simulink model "sim_BTMS"  (R2022b)
settings: Solver=FixedStepAuto  StartTime=0.0  StopTime=SimPara.t_sim  FixedStep=0.001  RelTol=1e-3
values from neighbouring files (symbols this model uses):
  BatPara = get_BatPara(BatPara, config_battery)    [sim_BTMS_interface.m]
  p = epe_mod(jj).p    [main_sim_BTMS_1_system_setup.m]
  SysPara = rmfield(SysPara, {'p','s'})    [main_sim_BTMS_1_system_setup.m]
undefined symbols (not defined in the file or in its folder): A, BTMSConfig, i, LSAPara, SimPara, x2_cal, x3_cal, x_cal
libraries: simulink x14, dspstat3 x7, dspindex x1
(part 3 of 4)

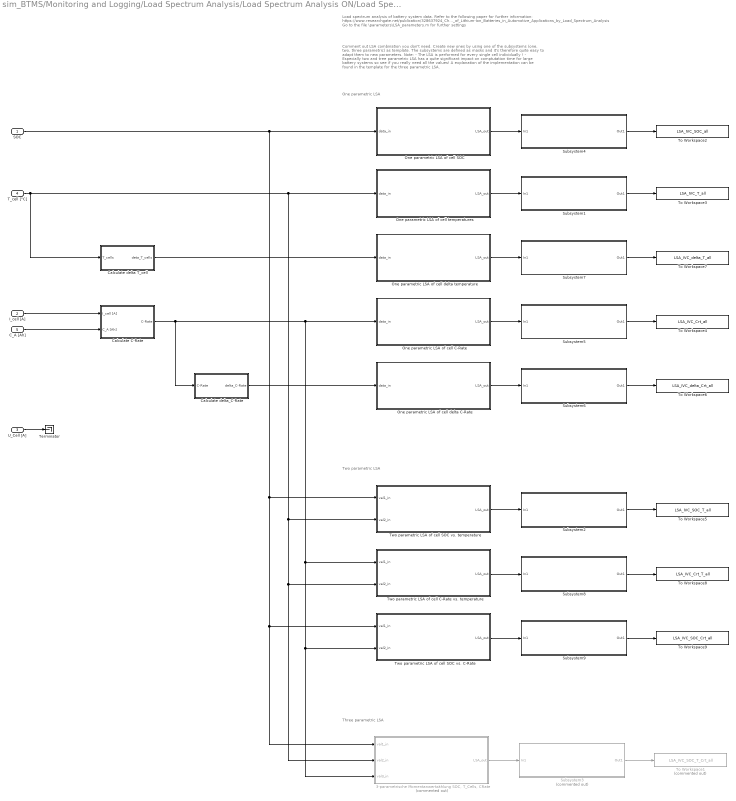
== system sim_BTMS/Monitoring and Logging/Load Spectrum Analysis/Load Spectrum Analysis ON/Load Spectrum Analysis ON ==
  note: Comment out LSA combination you don't need. Create new ones by using one of the subsystems (one, two, three parametric) as template. The subsystems are defined as masks
      | and it's therefore quite easy to adapt them to new parameters.
      |
      | Note:
      | - The LSA is performed for every single cell individually !
      | - Especially two and tree parametric LSA has a quite significant impact on comptutation time for large battery systems so see if you really need all the values!
      |
      | A explanation of the implementation can be found in the template for the three parametric LSA.
  note: Three parametric LSA
  note: Two parametric LSA
  note: One parametric LSA
  note: Load spectrum analysis of battery system data. Refer to the following paper for further information:
      | https://www.researchgate.net/publication/328637924_Characterization_and_Concept_Validation_of_Lithium-Ion_Batteries_in_Automotive_Applications_by_Load_Spectrum_Analysis
      |
      | Go to the file \parameters\LSA_parameters.m for further settings
  SOC : Inport
  I_cell [A] : Inport  Port=2
  U_Cell [A] : Inport  Port=3
  T_cell [°C] : Inport  Port=4
  C_A [Ah] : Inport  Port=5
  "3-parametrische Momentanwertzählung SOC, T_Cells, CRate" : Subsystem  Commented=on  mask{bins_borders_1=LSAPara.bins_borders_SOC, bins_mean_1=LSAPara.bins_mean_SOC, bins_borders_2=LSAPara.bins_borders_T, bins_mean_2=LSAPara.bins_mean_T, bins_borders_3=LSAPara.bins_borders_Crt, bins_mean_3=LSAPara.bins_mean_Crt}
      mask prompts: bins_borders_1 "Provide 'bins_borders'"; bins_mean_1 "Provide 'bins_mean'"; bins_borders_2 "Provide 'bins_borders'"; bins_mean_2 "Provide 'bins_mean'"; bins_borders_3 "Provide 'bins_borders'"; bins_mean_3 "Provide 'bins_mean'"
      mask DialogControl DescTextVar Prompt: Subsystem for three-parametric instantaneous value counting. Change the parameters below to select other system variables. Refer to parameters\LSA_parameters.m for further options.
      mask DialogControl Control2 Prompt: Copy&Paste this subsystem and double click to edit the variable assignments to monitor further variables.
      mask DialogControl Control3 Prompt: First system variable ('val 1')
      mask DialogControl Control4 Prompt: First system variable ('val 2')
      mask DialogControl Control5 Prompt: First system variable ('val 3')
      mask Display:
      | fprintf('Three parametric\ninstantaneous value\ncounting')
      | port_label('output', 1, 'load spectrum')
      | port_label('input', 1, 'timeseries val 1')
      | port_label('input', 2, 'timeseries val 2')
      | port_label('input', 3, 'timeseries val 3')
  Calculate C-Rate : Subsystem
  Calculate delta T_cell : Subsystem
  Calculate delta_C-Rate : Subsystem
  One parametric LSA of cell C-Rate : Subsystem  mask{bins_borders=LSAPara.bins_borders_Crt, bins_mean=LSAPara.bins_mean_Crt}
      mask prompts: bins_borders "Provide 'bins_borders'"; bins_mean "Provide 'bins_mean'"
      mask DialogControl DescTextVar Prompt: Subsystem for one-parametric instantaneous value counting. Change the parameters below to select other system variables. Refer to parameters\LSA_parameters.m for further options.
      mask DialogControl Control2 Prompt: Copy&Paste this subsystem and double click to edit the variable assignments to monitor further variables.
      mask Display:
      | fprintf('One parametric\ninstantaneous value\ncounting')
      | port_label('output', 1, 'load spectrum')
      | port_label('input', 1, 'timeseries')
  One parametric LSA of cell SOC : Subsystem  mask{bins_borders=LSAPara.bins_borders_SOC, bins_mean=LSAPara.bins_mean_SOC}
      mask prompts: bins_borders "Provide 'bins_borders'"; bins_mean "Provide 'bins_mean'"
      mask DialogControl DescTextVar Prompt: Subsystem for one-parametric instantaneous value counting. Change the parameters below to select other system variables. Refer to parameters\LSA_parameters.m for further options.
      mask DialogControl Control2 Prompt: Copy&Paste this subsystem and double click to edit the variable assignments to monitor further variables.
      mask Display:
      | fprintf('One parametric\ninstantaneous value\ncounting')
      | port_label('output', 1, 'load spectrum')
      | port_label('input', 1, 'timeseries')
  One parametric LSA of cell delta C-Rate : Subsystem  mask{bins_borders=LSAPara.bins_borders_delta_Crt, bins_mean=LSAPara.bins_mean_delta_Crt}
      mask prompts: bins_borders "Provide 'bins_borders'"; bins_mean "Provide 'bins_mean'"
      mask DialogControl DescTextVar Prompt: Subsystem for one-parametric instantaneous value counting. Change the parameters below to select other system variables. Refer to parameters\LSA_parameters.m for further options.
      mask DialogControl Control2 Prompt: Copy&Paste this subsystem and double click to edit the variable assignments to monitor further variables.
      mask Display:
      | fprintf('One parametric\ninstantaneous value\ncounting')
      | port_label('output', 1, 'load spectrum')
      | port_label('input', 1, 'timeseries')
  One parametric LSA of cell delta temperature : Subsystem  mask{bins_borders=LSAPara.bins_borders_delta_T, bins_mean=LSAPara.bins_mean_delta_T}
      mask prompts: bins_borders "Provide 'bins_borders'"; bins_mean "Provide 'bins_mean'"
      mask DialogControl DescTextVar Prompt: Subsystem for one-parametric instantaneous value counting. Change the parameters below to select other system variables. Refer to parameters\LSA_parameters.m for further options.
      mask DialogControl Control2 Prompt: Copy&Paste this subsystem and double click to edit the variable assignments to monitor further variables.
      mask Display:
      | fprintf('One parametric\ninstantaneous value\ncounting')
      | port_label('output', 1, 'load spectrum')
      | port_label('input', 1, 'timeseries')
  One parametric LSA of cell temperatures : Subsystem  mask{bins_borders=LSAPara.bins_borders_T, bins_mean=LSAPara.bins_mean_T}
      mask prompts: bins_borders "Provide 'bins_borders'"; bins_mean "Provide 'bins_mean'"
      mask DialogControl DescTextVar Prompt: Subsystem for one-parametric instantaneous value counting. Change the parameters below to select other system variables. Refer to parameters\LSA_parameters.m for further options.
      mask DialogControl Control2 Prompt: Copy&Paste this subsystem and double click to edit the variable assignments to monitor further variables.
      mask Display:
      | fprintf('One parametric\ninstantaneous value\ncounting')
      | port_label('output', 1, 'load spectrum')
      | port_label('input', 1, 'timeseries')
  Subsystem1 : Subsystem  mask{dim=2, start=99}
      mask prompts: dim "Select dimension"; start "Start concatenation after x%"
      mask DialogControl DescTextVar Prompt: Create one load spectrum from all individual cells. By default the LSA blocks create one load spectrum for every individual cell. This block creates one load-spectrum for all cells.
      mask DialogControl Control2 Prompt: Select the dimension of the load spectum in the parameter below. This uses the following logic:
      mask DialogControl Control3 Prompt: One parametric LS: Select "2"
      mask DialogControl Control4 Prompt: Two parametric LS: Select "3"
      mask DialogControl Control5 Prompt: Three parametric LS: Select "4"
      mask DialogControl Control6 Prompt: Only the last value of the load spectrum matrix is relevant, so we don't want to make the concatenation every simulation step. Therefore the system is set to only start with the calculation after 99% of the simulation is finished. If you need another value edit ist below.
      mask Display:
      | fprintf('Summed LSA\nfrom all cells')
      | port_label('input', 1, 'cell-individual LSA')
      | port_label('output', 1, 'summed LSA')
  Subsystem2 : Subsystem  mask{dim=3, start=99}
      mask prompts: dim "Select dimension"; start "Start concatenation after x%"
      mask DialogControl DescTextVar Prompt: Create one load spectrum from all individual cells. By default the LSA blocks create one load spectrum for every individual cell. This block creates one load-spectrum for all cells.
      mask DialogControl Control2 Prompt: Select the dimension of the load spectum in the parameter below. This uses the following logic:
      mask DialogControl Control3 Prompt: One parametric LS: Select "2"
      mask DialogControl Control4 Prompt: Two parametric LS: Select "3"
      mask DialogControl Control5 Prompt: Three parametric LS: Select "4"
      mask DialogControl Control6 Prompt: Only the last value of the load spectrum matrix is relevant, so we don't want to make the concatenation every simulation step. Therefore the system is set to only start with the calculation after 99% of the simulation is finished. If you need another value edit ist below.
      mask Display:
      | fprintf('Summed LSA\nfrom all cells')
      | port_label('input', 1, 'cell-individual LSA')
      | port_label('output', 1, 'summed LSA')
  Subsystem3 : Subsystem  Commented=on  mask{dim=4, start=99}
      mask prompts: dim "Select dimension"; start "Start concatenation after x%"
      mask DialogControl DescTextVar Prompt: Create one load spectrum from all individual cells. By default the LSA blocks create one load spectrum for every individual cell. This block creates one load-spectrum for all cells.
      mask DialogControl Control2 Prompt: Select the dimension of the load spectum in the parameter below. This uses the following logic:
      mask DialogControl Control3 Prompt: One parametric LS: Select "2"
      mask DialogControl Control4 Prompt: Two parametric LS: Select "3"
      mask DialogControl Control5 Prompt: Three parametric LS: Select "4"
      mask DialogControl Control6 Prompt: Only the last value of the load spectrum matrix is relevant, so we don't want to make the concatenation every simulation step. Therefore the system is set to only start with the calculation after 99% of the simulation is finished. If you need another value edit ist below.
      mask Display:
      | fprintf('Summed LSA\nfrom all cells')
      | port_label('input', 1, 'cell-individual LSA')
      | port_label('output', 1, 'summed LSA')
  Subsystem4 : Subsystem  mask{dim=2, start=99}
      mask prompts: dim "Select dimension"; start "Start concatenation after x%"
      mask DialogControl DescTextVar Prompt: Create one load spectrum from all individual cells. By default the LSA blocks create one load spectrum for every individual cell. This block creates one load-spectrum for all cells.
      mask DialogControl Control2 Prompt: Select the dimension of the load spectum in the parameter below. This uses the following logic:
      mask DialogControl Control3 Prompt: One parametric LS: Select "2"
      mask DialogControl Control4 Prompt: Two parametric LS: Select "3"
      mask DialogControl Control5 Prompt: Three parametric LS: Select "4"
      mask DialogControl Control6 Prompt: Only the last value of the load spectrum matrix is relevant, so we don't want to make the concatenation every simulation step. Therefore the system is set to only start with the calculation after 99% of the simulation is finished. If you need another value edit ist below.
      mask Display:
      | fprintf('Summed LSA\nfrom all cells')
      | port_label('input', 1, 'cell-individual LSA')
      | port_label('output', 1, 'summed LSA')
  Subsystem5 : Subsystem  mask{dim=2, start=99}
      mask prompts: dim "Select dimension"; start "Start concatenation after x%"
      mask DialogControl DescTextVar Prompt: Create one load spectrum from all individual cells. By default the LSA blocks create one load spectrum for every individual cell. This block creates one load-spectrum for all cells.
      mask DialogControl Control2 Prompt: Select the dimension of the load spectum in the parameter below. This uses the following logic:
      mask DialogControl Control3 Prompt: One parametric LS: Select "2"
      mask DialogControl Control4 Prompt: Two parametric LS: Select "3"
      mask DialogControl Control5 Prompt: Three parametric LS: Select "4"
      mask DialogControl Control6 Prompt: Only the last value of the load spectrum matrix is relevant, so we don't want to make the concatenation every simulation step. Therefore the system is set to only start with the calculation after 99% of the simulation is finished. If you need another value edit ist below.
      mask Display:
      | fprintf('Summed LSA\nfrom all cells')
      | port_label('input', 1, 'cell-individual LSA')
      | port_label('output', 1, 'summed LSA')
  Subsystem6 : Subsystem  mask{dim=2, start=99}
      mask prompts: dim "Select dimension"; start "Start concatenation after x%"
      mask DialogControl DescTextVar Prompt: Create one load spectrum from all individual cells. By default the LSA blocks create one load spectrum for every individual cell. This block creates one load-spectrum for all cells.
      mask DialogControl Control2 Prompt: Select the dimension of the load spectum in the parameter below. This uses the following logic:
      mask DialogControl Control3 Prompt: One parametric LS: Select "2"
      mask DialogControl Control4 Prompt: Two parametric LS: Select "3"
      mask DialogControl Control5 Prompt: Three parametric LS: Select "4"
      mask DialogControl Control6 Prompt: Only the last value of the load spectrum matrix is relevant, so we don't want to make the concatenation every simulation step. Therefore the system is set to only start with the calculation after 99% of the simulation is finished. If you need another value edit ist below.
      mask Display:
      | fprintf('Summed LSA\nfrom all cells')
      | port_label('input', 1, 'cell-individual LSA')
      | port_label('output', 1, 'summed LSA')
  Subsystem7 : Subsystem  mask{dim=2, start=99}
      mask prompts: dim "Select dimension"; start "Start concatenation after x%"
      mask DialogControl DescTextVar Prompt: Create one load spectrum from all individual cells. By default the LSA blocks create one load spectrum for every individual cell. This block creates one load-spectrum for all cells.
      mask DialogControl Control2 Prompt: Select the dimension of the load spectum in the parameter below. This uses the following logic:
      mask DialogControl Control3 Prompt: One parametric LS: Select "2"
      mask DialogControl Control4 Prompt: Two parametric LS: Select "3"
      mask DialogControl Control5 Prompt: Three parametric LS: Select "4"
      mask DialogControl Control6 Prompt: Only the last value of the load spectrum matrix is relevant, so we don't want to make the concatenation every simulation step. Therefore the system is set to only start with the calculation after 99% of the simulation is finished. If you need another value edit ist below.
      mask Display:
      | fprintf('Summed LSA\nfrom all cells')
      | port_label('input', 1, 'cell-individual LSA')
      | port_label('output', 1, 'summed LSA')
  Subsystem8 : Subsystem  mask{dim=3, start=99}
      mask prompts: dim "Select dimension"; start "Start concatenation after x%"
      mask DialogControl DescTextVar Prompt: Create one load spectrum from all individual cells. By default the LSA blocks create one load spectrum for every individual cell. This block creates one load-spectrum for all cells.
      mask DialogControl Control2 Prompt: Select the dimension of the load spectum in the parameter below. This uses the following logic:
      mask DialogControl Control3 Prompt: One parametric LS: Select "2"
      mask DialogControl Control4 Prompt: Two parametric LS: Select "3"
      mask DialogControl Control5 Prompt: Three parametric LS: Select "4"
      mask DialogControl Control6 Prompt: Only the last value of the load spectrum matrix is relevant, so we don't want to make the concatenation every simulation step. Therefore the system is set to only start with the calculation after 99% of the simulation is finished. If you need another value edit ist below.
      mask Display:
      | fprintf('Summed LSA\nfrom all cells')
      | port_label('input', 1, 'cell-individual LSA')
      | port_label('output', 1, 'summed LSA')
  Subsystem9 : Subsystem  mask{dim=3, start=99}
      mask prompts: dim "Select dimension"; start "Start concatenation after x%"
      mask DialogControl DescTextVar Prompt: Create one load spectrum from all individual cells. By default the LSA blocks create one load spectrum for every individual cell. This block creates one load-spectrum for all cells.
      mask DialogControl Control2 Prompt: Select the dimension of the load spectum in the parameter below. This uses the following logic:
      mask DialogControl Control3 Prompt: One parametric LS: Select "2"
      mask DialogControl Control4 Prompt: Two parametric LS: Select "3"
      mask DialogControl Control5 Prompt: Three parametric LS: Select "4"
      mask DialogControl Control6 Prompt: Only the last value of the load spectrum matrix is relevant, so we don't want to make the concatenation every simulation step. Therefore the system is set to only start with the calculation after 99% of the simulation is finished. If you need another value edit ist below.
      mask Display:
      | fprintf('Summed LSA\nfrom all cells')
      | port_label('input', 1, 'cell-individual LSA')
      | port_label('output', 1, 'summed LSA')
  Terminator : Terminator
  To Workspace1 : ToWorkspace  Commented=on  VariableName=LSA_IVC_SOC_T_Crt_all  SampleTime=-1
      settings: MaxDataPoints=1
  To Workspace2 : ToWorkspace  VariableName=LSA_IVC_SOC_all  SampleTime=-1
      settings: MaxDataPoints=1
  To Workspace3 : ToWorkspace  VariableName=LSA_IVC_T_all  SampleTime=-1
      settings: MaxDataPoints=1
  To Workspace4 : ToWorkspace  VariableName=LSA_IVC_Crt_all  SampleTime=-1
      settings: MaxDataPoints=1
  To Workspace5 : ToWorkspace  VariableName=LSA_IVC_SOC_T_all  SampleTime=-1
      settings: MaxDataPoints=1
  To Workspace6 : ToWorkspace  VariableName=LSA_IVC_delta_Crt_all  SampleTime=-1
      settings: MaxDataPoints=1
  To Workspace7 : ToWorkspace  VariableName=LSA_IVC_delta_T_all  SampleTime=-1
      settings: MaxDataPoints=1
  To Workspace8 : ToWorkspace  VariableName=LSA_IVC_Crt_T_all  SampleTime=-1
      settings: MaxDataPoints=1
  To Workspace9 : ToWorkspace  VariableName=LSA_IVC_SOC_Crt_all  SampleTime=-1
      settings: MaxDataPoints=1
  Two parametric LSA of cell C-Rate vs. temperature : Subsystem  mask{bins_borders_1=LSAPara.bins_borders_Crt, bins_mean_1=LSAPara.bins_mean_Crt, bins_borders_2=LSAPara.bins_borders_T, bins_mean_2=LSAPara.bins_mean_T}
      mask prompts: bins_borders_1 "Provide 'bins_borders'"; bins_mean_1 "Provide 'bins_mean'"; bins_borders_2 "Provide 'bins_borders'"; bins_mean_2 "Provide 'bins_mean'"
      mask DialogControl DescTextVar Prompt: Subsystem for twp-parametric instantaneous value counting. Change the parameters below to select other system variables. Refer to parameters\LSA_parameters.m for further options.
      mask DialogControl Control2 Prompt: Copy&Paste this subsystem and double click to edit the variable assignments to monitor further variables.
      mask DialogControl Control3 Prompt: First system variable ('val 1')
      mask DialogControl Control4 Prompt: Second system variable ('val 2')
      mask Display:
      | fprintf('Two parametric\ninstantaneous value\ncounting')
      | port_label('output', 1, 'load spectrum')
      | port_label('input', 1, 'timeseries val 1')
      | port_label('input', 2, 'timeseries val 2')
  Two parametric LSA of cell SOC vs. C-Rate : Subsystem  mask{bins_borders_1=LSAPara.bins_borders_SOC, bins_mean_1=LSAPara.bins_mean_SOC, bins_borders_2=LSAPara.bins_borders_Crt, bins_mean_2=LSAPara.bins_mean_Crt}
      mask prompts: bins_borders_1 "Provide 'bins_borders'"; bins_mean_1 "Provide 'bins_mean'"; bins_borders_2 "Provide 'bins_borders'"; bins_mean_2 "Provide 'bins_mean'"
      mask DialogControl DescTextVar Prompt: Subsystem for twp-parametric instantaneous value counting. Change the parameters below to select other system variables. Refer to parameters\LSA_parameters.m for further options.
      mask DialogControl Control2 Prompt: Copy&Paste this subsystem and double click to edit the variable assignments to monitor further variables.
      mask DialogControl Control3 Prompt: First system variable ('val 1')
      mask DialogControl Control4 Prompt: Second system variable ('val 2')
      mask Display:
      | fprintf('Two parametric\ninstantaneous value\ncounting')
      | port_label('output', 1, 'load spectrum')
      | port_label('input', 1, 'timeseries val 1')
      | port_label('input', 2, 'timeseries val 2')
  "Two parametric LSA of cell SOC vs. temperature " : Subsystem  mask{bins_borders_1=LSAPara.bins_borders_SOC, bins_mean_1=LSAPara.bins_mean_SOC, bins_borders_2=LSAPara.bins_borders_T, bins_mean_2=LSAPara.bins_mean_T}
      mask prompts: bins_borders_1 "Provide 'bins_borders'"; bins_mean_1 "Provide 'bins_mean'"; bins_borders_2 "Provide 'bins_borders'"; bins_mean_2 "Provide 'bins_mean'"
      mask DialogControl DescTextVar Prompt: Subsystem for twp-parametric instantaneous value counting. Change the parameters below to select other system variables. Refer to parameters\LSA_parameters.m for further options.
      mask DialogControl Control2 Prompt: Copy&Paste this subsystem and double click to edit the variable assignments to monitor further variables.
      mask DialogControl Control3 Prompt: First system variable ('val 1')
      mask DialogControl Control4 Prompt: Second system variable ('val 2')
      mask Display:
      | fprintf('Two parametric\ninstantaneous value\ncounting')
      | port_label('output', 1, 'load spectrum')
      | port_label('input', 1, 'timeseries val 1')
      | port_label('input', 2, 'timeseries val 2')
  wires:
  I_cell [A]/1 -> Calculate C-Rate/1(I_cell [A])
  SOC/1 -> "3-parametrische Momentanwertzählung SOC, T_Cells, CRate"/1(val1_in), Two parametric LSA of cell SOC vs. C-Rate/1(val1_in), "Two parametric LSA of cell SOC vs. temperature "/1(val1_in), One parametric LSA of cell SOC/1(data_in)
  C_A [Ah]/1 -> Calculate C-Rate/2(C_A [Ah])
  Calculate C-Rate/1(C-Rate) -> Calculate delta_C-Rate/1(C-Rate), One parametric LSA of cell C-Rate/1(data_in), "3-parametrische Momentanwertzählung SOC, T_Cells, CRate"/3(val3_in), Two parametric LSA of cell SOC vs. C-Rate/2(val2_in), Two parametric LSA of cell C-Rate vs. temperature/1(val1_in)
  "3-parametrische Momentanwertzählung SOC, T_Cells, CRate"/1(LSA_out) -> Subsystem3/1(In1)
  Subsystem1/1(Out1) -> To Workspace3/1
  One parametric LSA of cell temperatures/1(LSA_out) -> Subsystem1/1(In1)
  "Two parametric LSA of cell SOC vs. temperature "/1(LSA_out) -> Subsystem2/1(In1)
  Subsystem2/1(Out1) -> To Workspace5/1
  Subsystem3/1(Out1) -> To Workspace1/1
  U_Cell [A]/1 -> Terminator/1
  Calculate delta_C-Rate/1(delta_C-Rate) -> One parametric LSA of cell delta C-Rate/1(data_in)
  T_cell [°C]/1 -> Calculate delta T_cell/1(T_cells), One parametric LSA of cell temperatures/1(data_in), "3-parametrische Momentanwertzählung SOC, T_Cells, CRate"/2(val2_in), Two parametric LSA of cell C-Rate vs. temperature/2(val2_in), "Two parametric LSA of cell SOC vs. temperature "/2(val2_in)
  Calculate delta T_cell/1(deta_T_cells) -> One parametric LSA of cell delta temperature/1(data_in)
  Subsystem4/1(Out1) -> To Workspace2/1
  Subsystem5/1(Out1) -> To Workspace4/1
  Subsystem6/1(Out1) -> To Workspace6/1
  Subsystem7/1(Out1) -> To Workspace7/1
  One parametric LSA of cell SOC/1(LSA_out) -> Subsystem4/1(In1)
  One parametric LSA of cell C-Rate/1(LSA_out) -> Subsystem5/1(In1)
  One parametric LSA of cell delta C-Rate/1(LSA_out) -> Subsystem6/1(In1)
  One parametric LSA of cell delta temperature/1(LSA_out) -> Subsystem7/1(In1)
  Subsystem8/1(Out1) -> To Workspace8/1
  Subsystem9/1(Out1) -> To Workspace9/1
  Two parametric LSA of cell C-Rate vs. temperature/1(LSA_out) -> Subsystem8/1(In1)
  Two parametric LSA of cell SOC vs. C-Rate/1(LSA_out) -> Subsystem9/1(In1)

== system sim_BTMS/Monitoring and Logging/Temperature Sensor Simulation/Enable//disable temperature sensors/TempSensors OFF ==
  T_cell : Inport
  Constant : Constant  Value=0  OutDataTypeStr=boolean
  Terminator : Terminator
  T_sensors [°C] : Outport  VectorParamsAs1DForOutWhenUnconnected=off
  wires:
  T_cell/1 -> Terminator/1
  Constant/1 -> T_sensors [°C]/1  "T_sensors [°C]"

== system sim_BTMS/Monitoring and Logging/Temperature Sensor Simulation/Enable//disable temperature sensors/TempSensors ON ==
  T_cell : Inport
  Iterate through the sensors : Subsystem  TreatAsAtomicUnit=on
  Matrix to vector : Reshape  OutputDimensionality=Column vector (2-D)
  T_sensors [°C] : Outport  VectorParamsAs1DForOutWhenUnconnected=off
  wires:
  Matrix to vector/1 -> Iterate through the sensors/1(T_cells_vec)
  T_cell/1 -> Matrix to vector/1
  Iterate through the sensors/1(T_sensors [°C]) -> T_sensors [°C]/1  "T_sensors [°C]"

== system sim_BTMS/Battery system simulation/Thermal Submodel/Cell heat transport and heat dissipation/Heat transfer between cells/Heat transfer model switched OFF ==
  note: Heat transfer model switched off.
      | No heat transfer.
  T_cell_in : Inport
  Constant : Constant  Value=0
  Terminator1 : Terminator
  PQ_transfer : Outport  VectorParamsAs1DForOutWhenUnconnected=off
  wires:
  T_cell_in/1 -> Terminator1/1
  Constant/1 -> PQ_transfer/1  "PQ_transfer [W]"

== system sim_BTMS/Battery system simulation/Thermal Submodel/Cell heat transport and heat dissipation/Heat transfer between cells/Heat transfer model switched ON ==
  note: Calculate the heat transfer between cells:
      | - Cells exchange heat via a heat transfer coefficient.
      | - Those are defined in the matrix K_transfer
      | -Example for cell 1 exchanging heat will cell i:
      | PQ_lambda_cell = sum((T_i-T_1)/K_transfer(i,1))
  note: PQ_lambda = K_transfer * T_cell_in
  note: Column vector --> Matrix
  note: Matrix --> column vector
  T_cell_in : Inport
  Constant : Constant  Value=SysPara.thermal.transfer.K_transfer
  Product : Product  Multiplication=Matrix(*)
  Reshape1 : Reshape  OutputDimensionality=Column vector (2-D)
  Reshape2 : Reshape  OutputDimensionality=Customize  OutputDimensions=[SysPara.p, SysPara.s]
  PQ_transfer : Outport  VectorParamsAs1DForOutWhenUnconnected=off
  wires:
  T_cell_in/1 -> Reshape1/1
  Reshape2/1 -> PQ_transfer/1  "PQ_transfer [W]"
  Reshape1/1 -> Product/2
  Product/1 -> Reshape2/1
  Constant/1 -> Product/1

== system sim_BTMS/Battery system simulation/Thermal Submodel/Cell heat transport and heat dissipation/Lumped mass thermal cell model/dt ==
  Clock : Clock
  Subtract : Sum  Inputs=+-
  Unit Delay : UnitDelay  SampleTime=-1  HasFrameUpgradeWarning=on
  dt [s] : Outport  VectorParamsAs1DForOutWhenUnconnected=off
  wires:
  Unit Delay/1 -> Subtract/2
  Clock/1 -> Unit Delay/1, Subtract/1
  Subtract/1 -> dt [s]/1

== system sim_BTMS/Monitoring and Logging/Load Spectrum Analysis/Load Spectrum Analysis ON/Load Spectrum Analysis ON/3-parametrische Momentanwertzählung SOC, T_Cells, CRate ==
  val1_in : Inport
  val2_in : Inport  Port=2
  val3_in : Inport  Port=3
  For Iterator val1 : Subsystem  TreatAsAtomicUnit=on
  delay for selector data input : UnitDelay  SampleTime=-1  HasFrameUpgradeWarning=on
  LSA_out : Outport  VectorParamsAs1DForOutWhenUnconnected=off
  wires:
  val3_in/1 -> For Iterator val1/3(val3_in)
  val2_in/1 -> For Iterator val1/2(val2_in)
  val1_in/1 -> For Iterator val1/1(val1_in)
  For Iterator val1/1(LSA_out) -> LSA_out/1, delay for selector data input/1
  delay for selector data input/1 -> For Iterator val1/4(data_in_delayed)

== system sim_BTMS/Monitoring and Logging/Load Spectrum Analysis/Load Spectrum Analysis ON/Load Spectrum Analysis ON/Calculate C-Rate ==
  note: Note: We calculate the C-Rate for each cell using each cell's individual C_A!
  I_cell [A] : Inport
  C_A [Ah] : Inport  Port=2
  I --> C-Rate : Product  Inputs=*/
  C-Rate : Outport  VectorParamsAs1DForOutWhenUnconnected=off
  wires:
  I --> C-Rate/1 -> C-Rate/1
  I_cell [A]/1 -> I --> C-Rate/1
  C_A [Ah]/1 -> I --> C-Rate/2

== system sim_BTMS/Monitoring and Logging/Load Spectrum Analysis/Load Spectrum Analysis ON/Load Spectrum Analysis ON/Calculate delta T_cell ==
  T_cells : Inport
  Add : Sum  Inputs=+-
  Minimum : dspstat3/Minimum  operation=minimum  fcn=Value  indexBase=One  operateOver=Entire input  Dimension=1  InputProcessing=Columns as channels (frame based)  reset=None  roiEnable=off  roiType=Rectangles  roiPortion=Entire ROI  roiOutput=Individual statistics for each ROI  roiFlag=off  roundingMode=Floor  overflowMode=off
  deta_T_cells : Outport  VectorParamsAs1DForOutWhenUnconnected=off
  wires:
  T_cells/1 -> Add/1, Minimum/1
  Add/1 -> deta_T_cells/1
  Minimum/1 -> Add/2

== system sim_BTMS/Monitoring and Logging/Load Spectrum Analysis/Load Spectrum Analysis ON/Load Spectrum Analysis ON/Calculate delta_C-Rate ==
  note: Calculate the delta_C-Rate for each cell in respect to the lowest absolute C-Rate in the system for each time-step.
  C-Rate : Inport
  Bildung Differenz : Sum  Inputs=+-
  Minimum1 : dspstat3/Minimum  operation=minimum  fcn=Value  indexBase=One  operateOver=Entire input  Dimension=1  InputProcessing=Columns as channels (frame based)  reset=None  roiEnable=off  roiType=Rectangles  roiPortion=Entire ROI  roiOutput=Individual statistics for each ROI  roiFlag=off  roundingMode=Floor  overflowMode=off
  Product : Product
  Sign : Signum
  always positve : Abs  SaturateOnIntegerOverflow=off
  delta_C-Rate : Outport  VectorParamsAs1DForOutWhenUnconnected=off
  wires:
  always positve/1 -> Minimum1/1
  Bildung Differenz/1 -> delta_C-Rate/1
  Sign/1 -> Product/1
  C-Rate/1 -> Bildung Differenz/1, Sign/1, always positve/1
  Minimum1/1 -> Product/2
  Product/1 -> Bildung Differenz/2

== system sim_BTMS/Monitoring and Logging/Load Spectrum Analysis/Load Spectrum Analysis ON/Load Spectrum Analysis ON/One parametric LSA of cell C-Rate ==
  data_in : Inport
  For Iterator val1 : Subsystem  TreatAsAtomicUnit=on
  delay for selector data input : UnitDelay  SampleTime=-1  HasFrameUpgradeWarning=on
  LSA_out : Outport  VectorParamsAs1DForOutWhenUnconnected=off
  wires:
  data_in/1 -> For Iterator val1/1(data_in)
  For Iterator val1/1(LSA_out) -> delay for selector data input/1, LSA_out/1
  delay for selector data input/1 -> For Iterator val1/2(data_in_delay)

== system sim_BTMS/Monitoring and Logging/Load Spectrum Analysis/Load Spectrum Analysis ON/Load Spectrum Analysis ON/One parametric LSA of cell SOC ==
  data_in : Inport
  For Iterator val1 : Subsystem  TreatAsAtomicUnit=on
  delay for selector data input : UnitDelay  SampleTime=-1  HasFrameUpgradeWarning=on
  LSA_out : Outport  VectorParamsAs1DForOutWhenUnconnected=off
  wires:
  delay for selector data input/1 -> For Iterator val1/2(data_in_delay)
  For Iterator val1/1(LSA_out) -> LSA_out/1, delay for selector data input/1
  data_in/1 -> For Iterator val1/1(data_in)

== system sim_BTMS/Monitoring and Logging/Load Spectrum Analysis/Load Spectrum Analysis ON/Load Spectrum Analysis ON/One parametric LSA of cell delta C-Rate ==
  data_in : Inport
  For Iterator val1 : Subsystem  TreatAsAtomicUnit=on
  delay for selector data input : UnitDelay  SampleTime=-1  HasFrameUpgradeWarning=on
  LSA_out : Outport  VectorParamsAs1DForOutWhenUnconnected=off
  wires:
  delay for selector data input/1 -> For Iterator val1/2(data_in_delay)
  For Iterator val1/1(LSA_out) -> LSA_out/1, delay for selector data input/1
  data_in/1 -> For Iterator val1/1(data_in)

== system sim_BTMS/Monitoring and Logging/Load Spectrum Analysis/Load Spectrum Analysis ON/Load Spectrum Analysis ON/One parametric LSA of cell delta temperature ==
  data_in : Inport
  For Iterator val1 : Subsystem  TreatAsAtomicUnit=on
  delay for selector data input : UnitDelay  SampleTime=-1  HasFrameUpgradeWarning=on
  LSA_out : Outport  VectorParamsAs1DForOutWhenUnconnected=off
  wires:
  data_in/1 -> For Iterator val1/1(data_in)
  For Iterator val1/1(LSA_out) -> delay for selector data input/1, LSA_out/1
  delay for selector data input/1 -> For Iterator val1/2(data_in_delay)

== system sim_BTMS/Monitoring and Logging/Load Spectrum Analysis/Load Spectrum Analysis ON/Load Spectrum Analysis ON/One parametric LSA of cell temperatures ==
  data_in : Inport
  For Iterator val1 : Subsystem  TreatAsAtomicUnit=on
  delay for selector data input : UnitDelay  SampleTime=-1  HasFrameUpgradeWarning=on
  LSA_out : Outport  VectorParamsAs1DForOutWhenUnconnected=off
  wires:
  data_in/1 -> For Iterator val1/1(data_in)
  For Iterator val1/1(LSA_out) -> delay for selector data input/1, LSA_out/1
  delay for selector data input/1 -> For Iterator val1/2(data_in_delay)

== system sim_BTMS/Monitoring and Logging/Load Spectrum Analysis/Load Spectrum Analysis ON/Load Spectrum Analysis ON/Subsystem1 ==
  In1 : Inport
  Clock : Clock
  Compare To Constant : simulink/Logic and Bit Operations/Compare To Constant  relop=>=  const=start/100 * SimPara.t_sim  OutDataTypeStr=boolean
  SubsyMMatrssdatrixm : Subsystem
  Out1 : Outport  VectorParamsAs1DForOutWhenUnconnected=off
  wires:
  Clock/1 -> Compare To Constant/1
  Compare To Constant/1 -> SubsyMMatrssdatrixm/Enable
  SubsyMMatrssdatrixm/1(Out1) -> Out1/1
  In1/1 -> SubsyMMatrssdatrixm/1(In1)

== system sim_BTMS/Monitoring and Logging/Load Spectrum Analysis/Load Spectrum Analysis ON/Load Spectrum Analysis ON/Subsystem2 ==
  In1 : Inport
  Clock : Clock
  Compare To Constant : simulink/Logic and Bit Operations/Compare To Constant  relop=>=  const=start/100 * SimPara.t_sim  OutDataTypeStr=boolean
  SubsyMMatrssdatrixm : Subsystem
  Out1 : Outport  VectorParamsAs1DForOutWhenUnconnected=off
  wires:
  In1/1 -> SubsyMMatrssdatrixm/1(In1)
  SubsyMMatrssdatrixm/1(Out1) -> Out1/1
  Compare To Constant/1 -> SubsyMMatrssdatrixm/Enable
  Clock/1 -> Compare To Constant/1

== system sim_BTMS/Monitoring and Logging/Load Spectrum Analysis/Load Spectrum Analysis ON/Load Spectrum Analysis ON/Subsystem3 ==
  In1 : Inport
  Clock : Clock
  Compare To Constant : simulink/Logic and Bit Operations/Compare To Constant  relop=>=  const=start/100 * SimPara.t_sim  OutDataTypeStr=boolean
  SubsyMMatrssdatrixm : Subsystem
  Out1 : Outport  VectorParamsAs1DForOutWhenUnconnected=off
  wires:
  Clock/1 -> Compare To Constant/1
  Compare To Constant/1 -> SubsyMMatrssdatrixm/Enable
  SubsyMMatrssdatrixm/1(Out1) -> Out1/1
  In1/1 -> SubsyMMatrssdatrixm/1(In1)

== system sim_BTMS/Monitoring and Logging/Load Spectrum Analysis/Load Spectrum Analysis ON/Load Spectrum Analysis ON/Subsystem4 ==
  In1 : Inport
  Clock : Clock
  Compare To Constant : simulink/Logic and Bit Operations/Compare To Constant  relop=>=  const=start/100 * SimPara.t_sim  OutDataTypeStr=boolean
  SubsyMMatrssdatrixm : Subsystem
  Out1 : Outport  VectorParamsAs1DForOutWhenUnconnected=off
  wires:
  In1/1 -> SubsyMMatrssdatrixm/1(In1)
  SubsyMMatrssdatrixm/1(Out1) -> Out1/1
  Compare To Constant/1 -> SubsyMMatrssdatrixm/Enable
  Clock/1 -> Compare To Constant/1

== system sim_BTMS/Monitoring and Logging/Load Spectrum Analysis/Load Spectrum Analysis ON/Load Spectrum Analysis ON/Subsystem5 ==
  In1 : Inport
  Clock : Clock
  Compare To Constant : simulink/Logic and Bit Operations/Compare To Constant  relop=>=  const=start/100 * SimPara.t_sim  OutDataTypeStr=boolean
  SubsyMMatrssdatrixm : Subsystem
  Out1 : Outport  VectorParamsAs1DForOutWhenUnconnected=off
  wires:
  Clock/1 -> Compare To Constant/1
  Compare To Constant/1 -> SubsyMMatrssdatrixm/Enable
  SubsyMMatrssdatrixm/1(Out1) -> Out1/1
  In1/1 -> SubsyMMatrssdatrixm/1(In1)

== system sim_BTMS/Monitoring and Logging/Load Spectrum Analysis/Load Spectrum Analysis ON/Load Spectrum Analysis ON/Subsystem6 ==
  In1 : Inport
  Clock : Clock
  Compare To Constant : simulink/Logic and Bit Operations/Compare To Constant  relop=>=  const=start/100 * SimPara.t_sim  OutDataTypeStr=boolean
  SubsyMMatrssdatrixm : Subsystem
  Out1 : Outport  VectorParamsAs1DForOutWhenUnconnected=off
  wires:
  In1/1 -> SubsyMMatrssdatrixm/1(In1)
  SubsyMMatrssdatrixm/1(Out1) -> Out1/1
  Compare To Constant/1 -> SubsyMMatrssdatrixm/Enable
  Clock/1 -> Compare To Constant/1

== system sim_BTMS/Monitoring and Logging/Load Spectrum Analysis/Load Spectrum Analysis ON/Load Spectrum Analysis ON/Subsystem7 ==
  In1 : Inport
  Clock : Clock
  Compare To Constant : simulink/Logic and Bit Operations/Compare To Constant  relop=>=  const=start/100 * SimPara.t_sim  OutDataTypeStr=boolean
  SubsyMMatrssdatrixm : Subsystem
  Out1 : Outport  VectorParamsAs1DForOutWhenUnconnected=off
  wires:
  Clock/1 -> Compare To Constant/1
  Compare To Constant/1 -> SubsyMMatrssdatrixm/Enable
  SubsyMMatrssdatrixm/1(Out1) -> Out1/1
  In1/1 -> SubsyMMatrssdatrixm/1(In1)

== system sim_BTMS/Monitoring and Logging/Load Spectrum Analysis/Load Spectrum Analysis ON/Load Spectrum Analysis ON/Subsystem8 ==
  In1 : Inport
  Clock : Clock
  Compare To Constant : simulink/Logic and Bit Operations/Compare To Constant  relop=>=  const=start/100 * SimPara.t_sim  OutDataTypeStr=boolean
  SubsyMMatrssdatrixm : Subsystem
  Out1 : Outport  VectorParamsAs1DForOutWhenUnconnected=off
  wires:
  Clock/1 -> Compare To Constant/1
  Compare To Constant/1 -> SubsyMMatrssdatrixm/Enable
  SubsyMMatrssdatrixm/1(Out1) -> Out1/1
  In1/1 -> SubsyMMatrssdatrixm/1(In1)

== system sim_BTMS/Monitoring and Logging/Load Spectrum Analysis/Load Spectrum Analysis ON/Load Spectrum Analysis ON/Subsystem9 ==
  In1 : Inport
  Clock : Clock
  Compare To Constant : simulink/Logic and Bit Operations/Compare To Constant  relop=>=  const=start/100 * SimPara.t_sim  OutDataTypeStr=boolean
  SubsyMMatrssdatrixm : Subsystem
  Out1 : Outport  VectorParamsAs1DForOutWhenUnconnected=off
  wires:
  In1/1 -> SubsyMMatrssdatrixm/1(In1)
  SubsyMMatrssdatrixm/1(Out1) -> Out1/1
  Compare To Constant/1 -> SubsyMMatrssdatrixm/Enable
  Clock/1 -> Compare To Constant/1

== system sim_BTMS/Monitoring and Logging/Load Spectrum Analysis/Load Spectrum Analysis ON/Load Spectrum Analysis ON/Two parametric LSA of cell C-Rate vs. temperature ==
  val1_in : Inport
  val2_in : Inport  Port=2
  For Iterator val1 : Subsystem  TreatAsAtomicUnit=on
  delay for selector data input : UnitDelay  SampleTime=-1  HasFrameUpgradeWarning=on
  LSA_out : Outport  VectorParamsAs1DForOutWhenUnconnected=off
  wires:
  val2_in/1 -> For Iterator val1/2(val_2_in)
  val1_in/1 -> For Iterator val1/1(val1_in)
  For Iterator val1/1(LSA_out) -> LSA_out/1, delay for selector data input/1
  delay for selector data input/1 -> For Iterator val1/3(data_in_delayed)

== system sim_BTMS/Monitoring and Logging/Load Spectrum Analysis/Load Spectrum Analysis ON/Load Spectrum Analysis ON/Two parametric LSA of cell SOC vs. C-Rate ==
  val1_in : Inport
  val2_in : Inport  Port=2
  For Iterator val1 : Subsystem  TreatAsAtomicUnit=on
  delay for selector data input : UnitDelay  SampleTime=-1  HasFrameUpgradeWarning=on
  LSA_out : Outport  VectorParamsAs1DForOutWhenUnconnected=off
  wires:
  delay for selector data input/1 -> For Iterator val1/3(data_in_delayed)
  For Iterator val1/1(LSA_out) -> delay for selector data input/1, LSA_out/1
  val1_in/1 -> For Iterator val1/1(val1_in)
  val2_in/1 -> For Iterator val1/2(val_2_in)

== system sim_BTMS/Monitoring and Logging/Load Spectrum Analysis/Load Spectrum Analysis ON/Load Spectrum Analysis ON/Two parametric LSA of cell SOC vs. temperature  ==
  val1_in : Inport
  val2_in : Inport  Port=2
  For Iterator val1 : Subsystem  TreatAsAtomicUnit=on
  delay for selector data input : UnitDelay  SampleTime=-1  HasFrameUpgradeWarning=on
  LSA_out : Outport  VectorParamsAs1DForOutWhenUnconnected=off
  wires:
  delay for selector data input/1 -> For Iterator val1/3(data_in_delayed)
  For Iterator val1/1(LSA_out) -> delay for selector data input/1, LSA_out/1
  val1_in/1 -> For Iterator val1/1(val1_in)
  val2_in/1 -> For Iterator val1/2(val_2_in)

== system sim_BTMS/Monitoring and Logging/Temperature Sensor Simulation/Enable//disable temperature sensors/TempSensors ON/Iterate through the sensors ==
  note: Save sensor value in vector
  note: Get T_cell values for sensor
  note: Exclude zeros
  note: Select row of sensor
  note: Matrix with cell IDs for each sensor
  T_cells_vec : Inport
  Assignment : Assignment  DiagnosticForDimensions=Warning  IndexOptions=Index vector (port)  Indices=Sensor1  OutputSizes=1
  Constant : Constant  Value=SysPara.thermal.sensors.sensor_mat  VectorParams1D=off
  Find Nonzero Elements : Find  NumberOfInputDimensions=3  IndexMode=Zero-based  ShowOutputForNonzeroInputValues=on
  For Iterator : ForIterator  IterationLimit=size(SysPara.thermal.sensors.sensor_mat,1)
  Mean : dspstat3/Mean  run=off  InputProcessing=Columns as channels (frame based)  reset_popup=None  directionMode=Entire input  dimension=1  roiEnable=off  roiType=Rectangles  roiPortion=Entire ROI  roiOutput=Individual statistics for each ROI  roiFlag=off  roundingMode=Floor  overflowMode=off  outputDataTypeStr=Inherit: Same as accumulator  outputMin=[]  outputMax=[]  outputLastDataTypeStr=Inherit: Same as accumulator
  Memory : Memory  InitialCondition=zeros(size(SysPara.thermal.sensors.sensor_mat,1),1)  InheritSampleTime=on
  Selector1 : Selector  NumberOfDimensions=2  InputPortWidth=sn  IndexOptions=Index vector (port),Select all  Indices=A(i),1  OutputSizes=1,1
  Selector2 : Selector  InputPortWidth=SysPara.p * SysPara.s  IndexOptions=Index vector (port)  Indices=[1 3]  OutputSizes=1
  Terminator : Terminator
  T_sensors [°C] : Outport  VectorParamsAs1DForOutWhenUnconnected=off
  wires:
  For Iterator/1 -> Selector1/2, Assignment/3
  T_cells_vec/1 -> Selector2/1
  Selector2/1 -> Mean/1
  Assignment/1 -> T_sensors [°C]/1, Memory/1
  Mean/1 -> Assignment/2
  Memory/1 -> Assignment/1
  Constant/1 -> Selector1/1
  Selector1/1 -> Find Nonzero Elements/1
  Find Nonzero Elements/2 -> Selector2/2
  Find Nonzero Elements/1 -> Terminator/1

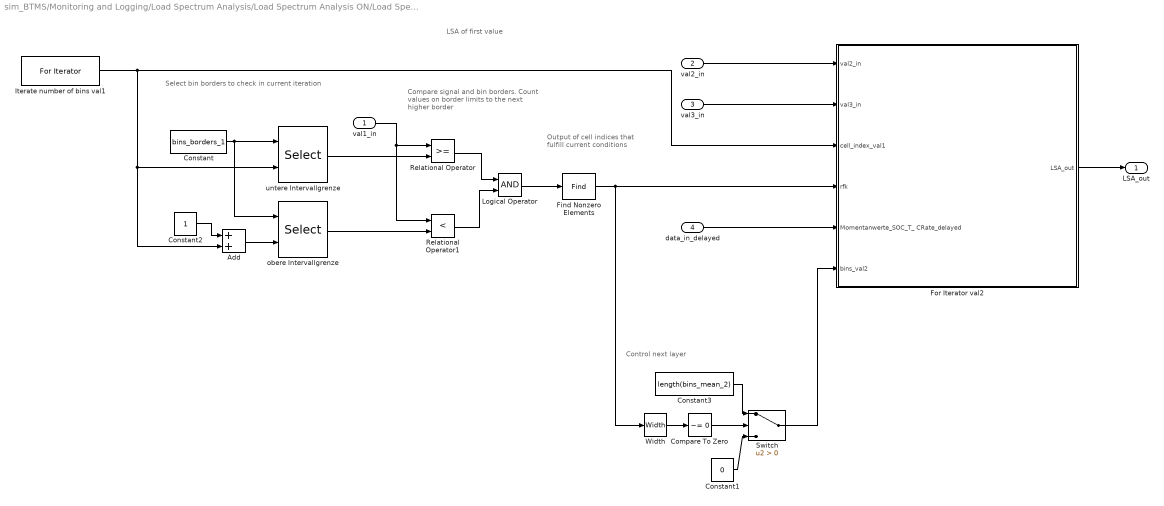
== system sim_BTMS/Monitoring and Logging/Load Spectrum Analysis/Load Spectrum Analysis ON/Load Spectrum Analysis ON/3-parametrische Momentanwertzählung SOC, T_Cells, CRate/For Iterator val1 ==
  note: Select bin borders to check in current iteration
  note: Output of cell indices that fulfill current conditions
  note: Compare signal and bin borders. Count values on border limits to the next higher border
  note: LSA of first value
  note: Control next layer
  val1_in : Inport
  val2_in : Inport  Port=2
  val3_in : Inport  Port=3
  data_in_delayed : Inport  Port=4
  Add : Sum
  Compare To Zero : simulink/Logic and Bit Operations/Compare To Zero  relop=~=  OutDataTypeStr=boolean
  Constant : Constant  Value=bins_borders_1
  Constant1 : Constant  Value=0
  Constant2 : Constant
  Constant3 : Constant  Value=length(bins_mean_2)
  Find Nonzero Elements : Find
  For Iterator val2 : Subsystem  TreatAsAtomicUnit=on
  Iterate number of bins val1 : ForIterator  ResetStates=reset  IterationLimit=length(bins_mean_1)  IterationVariableDataType=double
  Logical Operator : Logic  AllPortsSameDT=off  OutDataTypeStr=boolean
  Relational Operator : RelationalOperator  OutDataTypeStr=boolean  RndMeth=Simplest  InputSameDT=off
  Relational Operator1 : RelationalOperator  Operator=<  OutDataTypeStr=boolean  RndMeth=Simplest  InputSameDT=off
  Switch : Switch  Criteria=u2 > Threshold  SaturateOnIntegerOverflow=off  InputSameDT=off
  Width : Width
  obere Intervallgrenze : Selector  InputPortWidth=length(bins_borders_1)  IndexOptions=Index vector (port)  Indices=1:p  OutputSizes=1
  untere Intervallgrenze : Selector  InputPortWidth=length(bins_borders_1)  IndexOptions=Index vector (port)  Indices=1:p  OutputSizes=1
  LSA_out : Outport  VectorParamsAs1DForOutWhenUnconnected=off
  wires:
  Switch/1 -> For Iterator val2/6(bins_val2)
  Constant3/1 -> Switch/1
  Width/1 -> Compare To Zero/1
  Constant1/1 -> Switch/3
  Compare To Zero/1 -> Switch/2
  Find Nonzero Elements/1 -> For Iterator val2/4(rfk), Width/1
  val3_in/1 -> For Iterator val2/2(val3_in)
  val2_in/1 -> For Iterator val2/1(val2_in)
  Logical Operator/1 -> Find Nonzero Elements/1
  Relational Operator/1 -> Logical Operator/1
  Relational Operator1/1 -> Logical Operator/2
  val1_in/1 -> Relational Operator/1, Relational Operator1/1
  obere Intervallgrenze/1 -> Relational Operator1/2
  untere Intervallgrenze/1 -> Relational Operator/2
  Iterate number of bins val1/1 -> For Iterator val2/3(cell_index_val1), untere Intervallgrenze/2, Add/2
  Constant2/1 -> Add/1
  Add/1 -> obere Intervallgrenze/2
  Constant/1 -> untere Intervallgrenze/1, obere Intervallgrenze/1
  For Iterator val2/1(LSA_out) -> LSA_out/1
  data_in_delayed/1 -> For Iterator val2/5(Momentanwerte_SOC_T_ CRate_delayed)

== system sim_BTMS/Monitoring and Logging/Load Spectrum Analysis/Load Spectrum Analysis ON/Load Spectrum Analysis ON/One parametric LSA of cell C-Rate/For Iterator val1 ==
  data_in : Inport
  data_in_delay : Inport  Port=2
  Add : Sum
  Assignment Subsystem : Subsystem  TreatAsAtomicUnit=on
  Constant : Constant  Value=bins_borders
  Constant2 : Constant
  Find Nonzero Elements : Find
  Iterate number of bins : ForIterator  ResetStates=reset  IterationLimit=length(bins_mean)  IterationVariableDataType=double
  Logical Operator : Logic  AllPortsSameDT=off  OutDataTypeStr=boolean
  Relational Operator : RelationalOperator  OutDataTypeStr=boolean  RndMeth=Simplest  InputSameDT=off
  Relational Operator1 : RelationalOperator  Operator=<  OutDataTypeStr=boolean  RndMeth=Simplest  InputSameDT=off
  select bin upper border : Selector  InputPortWidth=length(bins_borders)  IndexOptions=Index vector (port)  Indices=1:p  OutputSizes=1
  select parallel cell2 : Selector  InputPortWidth=length(bins_borders)  IndexOptions=Index vector (port)  Indices=1:p  OutputSizes=1
  LSA_out : Outport  VectorParamsAs1DForOutWhenUnconnected=off
  wires:
  Assignment Subsystem/1(LSA_out) -> LSA_out/1
  Find Nonzero Elements/1 -> Assignment Subsystem/2(index_cell)
  Logical Operator/1 -> Find Nonzero Elements/1
  Relational Operator/1 -> Logical Operator/1
  Relational Operator1/1 -> Logical Operator/2
  data_in/1 -> Relational Operator/1, Relational Operator1/1
  select bin upper border/1 -> Relational Operator1/2
  select parallel cell2/1 -> Relational Operator/2
  Iterate number of bins/1 -> select parallel cell2/2, Assignment Subsystem/1(k), Add/2
  Constant2/1 -> Add/1
  Add/1 -> select bin upper border/2
  Constant/1 -> select parallel cell2/1, select bin upper border/1
  data_in_delay/1 -> Assignment Subsystem/3(data_in_delayed)

== system sim_BTMS/Monitoring and Logging/Load Spectrum Analysis/Load Spectrum Analysis ON/Load Spectrum Analysis ON/One parametric LSA of cell SOC/For Iterator val1 ==
  data_in : Inport
  data_in_delay : Inport  Port=2
  Add : Sum
  Assignment Subsystem : Subsystem  TreatAsAtomicUnit=on
  Constant : Constant  Value=bins_borders
  Constant2 : Constant
  Find Nonzero Elements : Find
  Iterate number of bins : ForIterator  ResetStates=reset  IterationLimit=length(bins_mean)  IterationVariableDataType=double
  Logical Operator : Logic  AllPortsSameDT=off  OutDataTypeStr=boolean
  Relational Operator : RelationalOperator  OutDataTypeStr=boolean  RndMeth=Simplest  InputSameDT=off
  Relational Operator1 : RelationalOperator  Operator=<  OutDataTypeStr=boolean  RndMeth=Simplest  InputSameDT=off
  select bin upper border : Selector  InputPortWidth=length(bins_borders)  IndexOptions=Index vector (port)  Indices=1:p  OutputSizes=1
  select parallel cell2 : Selector  InputPortWidth=length(bins_borders)  IndexOptions=Index vector (port)  Indices=1:p  OutputSizes=1
  LSA_out : Outport  VectorParamsAs1DForOutWhenUnconnected=off
  wires:
  data_in_delay/1 -> Assignment Subsystem/3(data_in_delayed)
  Constant/1 -> select bin upper border/1, select parallel cell2/1
  Add/1 -> select bin upper border/2
  Constant2/1 -> Add/1
  Iterate number of bins/1 -> Add/2, Assignment Subsystem/1(k), select parallel cell2/2
  select parallel cell2/1 -> Relational Operator/2
  select bin upper border/1 -> Relational Operator1/2
  data_in/1 -> Relational Operator1/1, Relational Operator/1
  Relational Operator1/1 -> Logical Operator/2
  Relational Operator/1 -> Logical Operator/1
  Logical Operator/1 -> Find Nonzero Elements/1
  Find Nonzero Elements/1 -> Assignment Subsystem/2(index_cell)
  Assignment Subsystem/1(LSA_out) -> LSA_out/1
